simulink model "BuildingHeatLoadCalc"  (R2026a)
settings: Solver=ode1be  StopTime=31532400  FixedStep=3600  AbsTol=1e-3
undefined symbols (not defined in the file): BuildingThermalLib, lib_BuildingThermal
libraries: ExternalWall_lib x47, WallSelector_lib x36, fl_lib x32, RoomWithAirVolume x15, nesl_utility x4, TemperatureSource_lib x1, DayScheduler_lib x1, SolarRadiationAtLocation_lib x1
(part 1 of 5)
settings Model: Creator=vikrants  LastModifiedBy=vikrants
settings DebuggingCC: SymbolicDimsDataTypeCodeGenerationDiagnostic=none
settings SimscapeCC: SimscapeNominalValues="[{\"value\":\"1\",\"unit\":\"A\"},{\"value\":\"1\",\"unit\":\"bar\"},{\"value\":\"1\",\"unit\":\"cm^2\"},{\"value\":\"1\",\"unit\":\"cm^3/s\"},{\"value\":\"1\",\"unit\":\"kJ/kg\"},{\"value\":\"1\",\"unit\":\"kW\"},{\"value\":\"1\",\"unit\":\"l\"},{\"value\":\"1\",\"unit\":\"N\"},{\"value\":\"1\",\"unit\":\"N*m\"},{\"value\":\"1\",\"unit\":\"V\"}]"  SimscapeLogSimulationStatistics=on

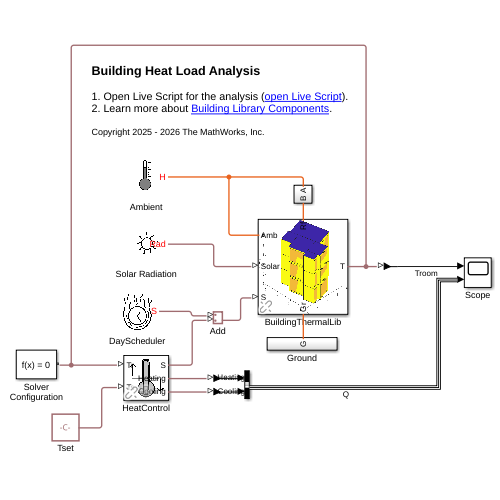
[thumbnail: Simulink's stored preview of the top-level diagram]
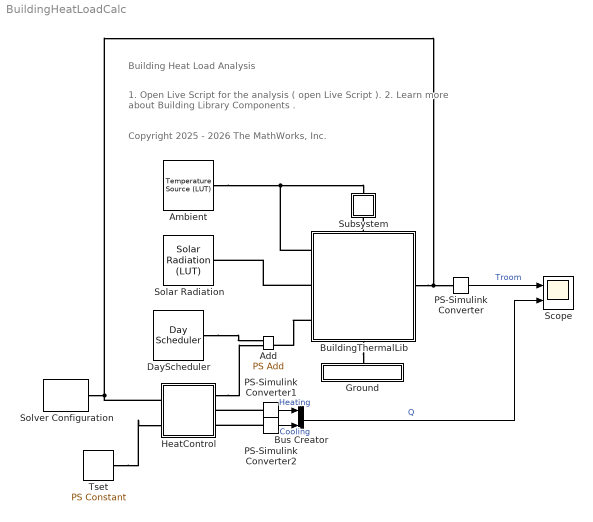
== system BuildingHeatLoadCalc ==
  note: Copyright 2025 - 2026 The MathWorks, Inc.
  note: Building Heat Load Analysis
  note: 1. Open Live Script for the analysis ( open Live Script ).
      | 2. Learn more about Building Library Components .
  Add : fl_lib/Physical Signals/Functions/PS Add
  Ambient : TemperatureSource_lib/Temperature Source (LUT)  latitude=47.376 % Parameterized on : 09-Jun-2026 19:38:28  longitude=8.541 % Parameterized on : 09-Jun-2026 19:38:29  localTime=15.00 % Parameterized on : 09-Jun-2026 19:38:29  dayLightS=0 % Parameterized on : 09-Jun-2026 19:38:29  startYear=2024 % Parameterized on : 09-Jun-2026 19:38:29  startMonth=1 % Parameterized on : 09-Jun-2026 19:38:29  startDay=1 % Parameterized on : 09-Jun-2026 19:38:29  startHr=1 % Parameterized on : 09-Jun-2026 19:38:29  numDaysData=365 % Parameterized on : 09-Jun-2026 19:38:29  interp_method=simscape.enum.interpolation.linear  extrap_method=simscape.enum.extrapolation.error  avgDayTvec="[275.3273      275.3222      275.3145      275.3043      275.2918      275.2771      275.3018      275.3282      275.3563      275.3861      275.4173        275.45      275.4841      275.5195      275.5562       275.594      275.6331      275.6733      275.7145      275.7568         275.8      275.8386      275.8744      275.9074      275.9378      275.9656       275.991      276.0141      276.0349      276.0536      276.0701      276.0846      276.0971      276.1078      276.1166      276.1236      276.1305      276.1619      276.1941      276.2271       276.261      276.2956      276.3309       276.367      276.4038      276.4412      276.4794      276.5181      276.5575      276.5975      276.6381      276.6792      276.7333       276.785      276.8342      276.9014      276.9656      277.0268      277.0851      277.1404      277.1927       277.242      277.2883      277.3317       277.372      277.4094      277.4438      277.4999       277.556      277.6119      277.6889      277.7686      277.8509      277.9359      278.0236       278.114       278.207      278.3028      278.4011      278.5022       278.606      278.7124      278.8297      278.9463      279.0624      279.1766      279.2694      279.3592      279.4459      279.5295      279.6101      279.6876      279.7621      279.8335      279.9018      279.9671      280.0294      280.0904      280.1795      280.2693      280.3596      280.4567      280.5571      280.6608      280.7677       280.878      280.9915      281.1083      281.2284      281.3518      281.4785      281.6085      281.7417      281.8694      281.9961      282.0985      282.1971      282.2917      282.3825      282.4693      282.5523      282.6313      282.7065      282.7778      282.8451      282.9086      282.9681      283.0238      283.1102       283.192      283.2729      283.3518      283.4287      283.5036      283.5765      283.6475      283.7164      283.7834      283.8484      283.9114      283.9724      284.0314      284.0885      284.1997      284.3147      284.4321      284.5312      284.6314      284.7328      284.8353       284.939      285.0438      285.1498      285.2569      285.3651      285.4745      285.5851      285.6968      285.8072      285.8771      285.9433      285.9937       286.043      286.0913      286.1386      286.1849      286.2303      286.2746       286.318      286.3603      286.4017       286.442      286.4814      286.5198      286.5795      286.6422      286.6832      286.7242      286.7654      286.8066      286.8479      286.8892      286.9307      286.9722      287.0138      287.0554      287.0972       287.139      287.1809      287.2213      287.2359      287.2392      287.2429      287.2469      287.2511      287.2557      287.2606      287.2658      287.2713      287.2771      287.2833      287.2897      287.2964      287.3034      287.3108      287.3141      287.3186      287.2947      287.2701      287.2447      287.2186      287.1917       287.164      287.1356      287.1063      287.0764      287.0456      287.0141      286.9819      286.9489      286.8969       286.842       286.793      286.7455      286.6993      286.6545      286.6111       286.569      286.5284      286.4891      286.4511      286.4146      286.3794      286.3456      286.3132      286.2703      286.2305      286.1593       286.092      286.0289      285.9698      285.9148      285.8638      285.8168      285.7739      285.7351      285.7003      285.6696      285.6429      285.6203      285.6009      285.5726      285.4907      285.4055      285.3171      285.2255      285.1307      285.0327      284.9315      284.8271      284.7194      284.6086      284.4945      284.3772      284.2567       284.133      283.9973      283.8627      283.7683      283.6776      283.5904      283.5067      283.4267      283.3502      283.2772      283.2078       283.142      283.0798      283.0212      282.9661      282.9145      282.8475      282.7818      282.6951      282.6058      282.5138 ...(+1106 chars)] % Parameterized on : 09-Jun-2026 19:38:29 K"  pcDayTvar=2 % Parameterized on : 09-Jun-2026 19:38:29  avgNightTvec="[270.3273      270.3222      270.3145      270.3043      270.2918      270.2771      270.3018      270.3282      270.3563      270.3861      270.4173        270.45      270.4841      270.5195      270.5562       270.594      270.6331      270.6733      270.7145      270.7568         270.8      270.8386      270.8744      270.9074      270.9378      270.9656       270.991      271.0141      271.0349      271.0536      271.0701      271.0846      271.0971      271.1078      271.1166      271.1236      271.1305      271.1619      271.1941      271.2271       271.261      271.2956      271.3309       271.367      271.4038      271.4412      271.4794      271.5181      271.5575      271.5975      271.6381      271.6792      271.7333       271.785      271.8342      271.9014      271.9656      272.0268      272.0851      272.1404      272.1927       272.242      272.2883      272.3317       272.372      272.4094      272.4438      272.4999       272.556      272.6119      272.6889      272.7686      272.8509      272.9359      273.0236       273.114       273.207      273.3028      273.4011      273.5022       273.606      273.7124      273.8297      273.9463      274.0624      274.1766      274.2694      274.3592      274.4459      274.5295      274.6101      274.6876      274.7621      274.8335      274.9018      274.9671      275.0294      275.0904      275.1795      275.2693      275.3596      275.4567      275.5571      275.6608      275.7677       275.878      275.9915      276.1083      276.2284      276.3518      276.4785      276.6085      276.7417      276.8694      276.9961      277.0985      277.1971      277.2917      277.3825      277.4693      277.5523      277.6313      277.7065      277.7778      277.8451      277.9086      277.9681      278.0238      278.1102       278.192      278.2729      278.3518      278.4287      278.5036      278.5765      278.6475      278.7164      278.7834      278.8484      278.9114      278.9724      279.0314      279.0885      279.1997      279.3147      279.4321      279.5312      279.6314      279.7328      279.8353       279.939      280.0438      280.1498      280.2569      280.3651      280.4745      280.5851      280.6968      280.8072      280.8771      280.9433      280.9937       281.043      281.0913      281.1386      281.1849      281.2303      281.2746       281.318      281.3603      281.4017       281.442      281.4814      281.5198      281.5795      281.6422      281.6832      281.7242      281.7654      281.8066      281.8479      281.8892      281.9307      281.9722      282.0138      282.0554      282.0972       282.139      282.1809      282.2213      282.2359      282.2392      282.2429      282.2469      282.2511      282.2557      282.2606      282.2658      282.2713      282.2771      282.2833      282.2897      282.2964      282.3034      282.3108      282.3141      282.3186      282.2947      282.2701      282.2447      282.2186      282.1917       282.164      282.1356      282.1063      282.0764      282.0456      282.0141      281.9819      281.9489      281.8969       281.842       281.793      281.7455      281.6993      281.6545      281.6111       281.569      281.5284      281.4891      281.4511      281.4146      281.3794      281.3456      281.3132      281.2703      281.2305      281.1593       281.092      281.0289      280.9698      280.9148      280.8638      280.8168      280.7739      280.7351      280.7003      280.6696      280.6429      280.6203      280.6009      280.5726      280.4907      280.4055      280.3171      280.2255      280.1307      280.0327      279.9315      279.8271      279.7194      279.6086      279.4945      279.3772      279.2567       279.133      278.9973      278.8627      278.7683      278.6776      278.5904      278.5067      278.4267      278.3502      278.2772      278.2078       278.142      278.0798      278.0212      277.9661      277.9145      277.8475      277.7818      277.6951      277.6058      277.5138 ...(+1106 chars)] % Parameterized on : 09-Jun-2026 19:38:29 K"  pcNightTvar=3 % Parameterized on : 09-Jun-2026 19:38:29
  BuildingThermalLib : Subsystem  AncestorBlock=lib_BuildingThermal/BuildingThermalLib
      settings: PortSchema="{\"entries\":[{\"content\":{\"sides\":[{\"content\":{\"connectorIds\":[\"LConn1\",\"LConn2\",\"LConn3\"]},\"type\":\"ConnectorPlacement.EquallySpacedRectSide\",\"uuid\":\"02f2e3a8-9f92-46e9-bc8d-cac18fd60cc5\"},{\"content\":{\"connectorIds\":[\"RConn1\"],\"side\":\"RIGHT\"},\"type\":\"ConnectorPlacement.EquallySpacedRectSide\",\"uuid\":\"8e7293df-d9e6-4251-9074-f41050b516bb\"},{\"content\":{\"connectorIds\":[\"LConn4\"],\"side\":\"TOP\"},\"type\":\"ConnectorPlacement.EquallySpacedRectSide\",\"uuid\":\"59004dc2-3d8b-47ae-86a8-cbcf5fc5c8f5\"},{\"content\":{\"connectorIds\":[\"RConn2\"],\"side\":\"BOTTOM\"},\"type\":\"ConnectorPlacement.EquallySpacedRectSide\",\"uuid\":\"040a7ff5-3de3-404c-857a-2e2aad7a1fa3\"}]},\"type\":\"ConnectorPlacement.EquallySpacedConnector\",\"uuid\":\"ad5b2bd3-ca1b-4c9b-b2dc-e1849bcec5d6\"}],\"packageUris\":[\"http://schema.mathworks.com/mf0/Connector/R2020b\"],\"version\":\"1.0\"}"
      mask Display: image('lib_BuildingThermal.png')
  Bus Creator : BusCreator  Inputs=2
  DayScheduler : DayScheduler_lib/Day Scheduler  numRoom=15 % Parameterized on : 09-Jun-2026 19:38:32  roomIndex=[1 2 3 4 5 6 7 8 9 10 11 12 13 14 15] % Parameterized on : 09-Jun-2026 19:38:32  heatSource=[0 0 0 0 0 0 0 0 0 0 0 0 0 0 0 0 0 0 0 0 0 0 0 0;200 200 200 200 200 200 0 0 0 0 0 0 0 0 0 0 0 0 0 200 200 200 200 200;0 0 0 0 0 300 300 0 0 0 0 0 0 0 0 0 0 300 300 300 300 0 0 0;0 0 0 0 0 0 0 0 0 0 0 0 0 0 0 0 0 0 0 0 0 0 0 0;0 0 0 0 0 0 0 0 0 0 0 0 0 0 0 0 0 0 0 0 0 0 0 0;0 0 0 0 0 0 0 0 0 0 0 0 0 0 0 0 0 0 0 0 0 0 0 0;200 200 200 200 200 200 0 0 0 0 0 0 0 0 0 0 0 0 0 200 200 200 200 200;0 0 0 0 0 300 300 0 0 0 0 0 0 0 0 0 0 300 300 300 300 0 0 0;0 0 0 0 0 0 0 0 0 0 0 0 0 0 0 0 0 0 0 0 0 0 0 0;0 0 0 0 0 0 0 0 0 0 0 0 0 0 0 0 0 0 0 0 0 0 0 0;0 0 0 0 0 0 0 0 0 0 0 0 0 0 0 0 0 0 0 0 0 0 0 0;200 200 200 200 200 200 0 0 0 0 0 0 0 0 0 0 0 0 0 200 200 200 200 200;0 0 0 0 0 300 300 0 0 0 0 0 0 0 0 0 0 300 300 300 300 0 0 0;0 0 0 0 0 0 0 0 0 0 0 0 0 0 0 0 0 0 0 0 0 0 0 0;0 0 0 0 0 0 0 0 0 0 0 0 0 0 0 0 0 0 0 0 0 0 0 0] % Parameterized on : 09-Jun-2026 19:38:32 W  t=1 : 24  oneHr=3600
  Ground : Subsystem
      settings: PortSchema="{\"entries\":[{\"content\":{\"sides\":[{\"content\":{},\"type\":\"ConnectorPlacement.EquallySpacedRectSide\",\"uuid\":\"0537d5ec-4a94-45e2-a0dd-9776fcfbef5c\"},{\"content\":{\"side\":\"RIGHT\"},\"type\":\"ConnectorPlacement.EquallySpacedRectSide\",\"uuid\":\"ea52c298-5a99-4146-b05a-e741d3f0a75b\"},{\"content\":{\"connectorIds\":[\"LConn1\"],\"side\":\"TOP\"},\"type\":\"ConnectorPlacement.EquallySpacedRectSide\",\"uuid\":\"d3185eb6-f3c0-4f94-b2cb-94c943d4e977\"}]},\"type\":\"ConnectorPlacement.EquallySpacedConnector\",\"uuid\":\"099be505-a3d7-43d0-9da6-14e4de4f60b9\"}],\"packageUris\":[\"http://schema.mathworks.com/mf0/Connector/R2020b\"],\"version\":\"1.0\"}"
  HeatControl : Subsystem  AncestorBlock=HeatSourceControl/Heat Source Control  mask{capacity=12000, num=3, delT=10, tau=1, iniT=280}
      mask prompts: capacity "Heat pump capacity (W)"; num "Number of sources (-)"; delT "Change in water temperature (deg C)"; tau "Measurement time constant (s)"; iniT "Initial water temperature (K)"
      mask DialogControl DescTextVar Prompt: Simple heat source pump based on temperature difference between measured and set point values. The pump is an abstract implementation for Air Water Heat Pump (AWHP).
      mask DialogControl HeatPump Prompt: Heat Pump
      mask Display: image('HeatSourceControlIcon.png');
  PS-Simulink Converter : nesl_utility/PS-Simulink Converter  PhysicalDomain=network_engine_domain  SubClassName=ps_output  LeftPortType=input  RightPortType=output  PseudoPeriodic=off  Frequencies=[]  VectorFormat=inherit  Unit=inherit  AffineConversion=off
  PS-Simulink Converter1 : nesl_utility/PS-Simulink Converter  PhysicalDomain=network_engine_domain  SubClassName=ps_output  LeftPortType=input  RightPortType=output  PseudoPeriodic=off  Frequencies=[]  VectorFormat=inherit  Unit=inherit  AffineConversion=off
  PS-Simulink Converter2 : nesl_utility/PS-Simulink Converter  PhysicalDomain=network_engine_domain  SubClassName=ps_output  LeftPortType=input  RightPortType=output  PseudoPeriodic=off  Frequencies=[]  VectorFormat=inherit  Unit=inherit  AffineConversion=off
  Scope : Scope  NumInputPorts=2
      settings: ActiveDisplayYMinimum=-1  ActiveDisplayYMaximum=1
  Solar Radiation : SolarRadiationAtLocation_lib/Solar Radiation (LUT)  latitude=47.376 % Parameterized on : 09-Jun-2026 19:38:30  longitude=8.541 % Parameterized on : 09-Jun-2026 19:38:30  localTime=15.00 % Parameterized on : 09-Jun-2026 19:38:30  dayLightS=0 % Parameterized on : 09-Jun-2026 19:38:31  startYear=2024 % Parameterized on : 09-Jun-2026 19:38:30  startMonth=1 % Parameterized on : 09-Jun-2026 19:38:31  startDay=1 % Parameterized on : 09-Jun-2026 19:38:31  startHr=1 % Parameterized on : 09-Jun-2026 19:38:31  numHrsData=8760 % Parameterized on : 09-Jun-2026 19:38:31  cloudData=cloudCoverLibOption.none  cloudCoverVal=zeros(1, 24)  interp_method=simscape.enum.interpolation.linear  extrap_method=simscape.enum.extrapolation.nearest
  Solver Configuration : nesl_utility/Solver Configuration  PhysicalDomain=network_engine_domain  SubClassName=solver  LeftPortType=input  RightPortType=generic  Tones=[]  Harmonics=[]  SimulateNoise=off  Profile=off  UseLocalSampling=off  EnableSwitchedLinearOptims=on  FrequencyDomain=off  UseCCode=off  RelTol=0.001  AbsTol=1e-06  MinStep=1e-09  ToWorkspace=off  RevertToSquareIcSolve=off  NumHomotopyIterations=100  PhasorMode=off  PhasorModeNumHarmonics=1  ConsistencySolver=NEWTON_XTOL_AFTER_FTOL  CanonicalOrdering=UNORDERED  OptimizeIntermediates=UNOPTIMIZED  IndexReductionMethod=DerivativeReplacement  DoDC=off  ResidualTolerance=1e-09  ConsistencyTolSource=GLOBAL  ConsistencyAbsTol=0.001  ConsistencyRelTol=0.001  ConsistencyTolFactor=0.001  UseLocalSolver=off  LocalSolverChoice=NE_BACKWARD_EULER_ADVANCER  ResolveIndetEquations=on  FunctionEvalNumThread=1  LocalSolverSampleTime=0.001  DoFixedCost=off  MaxNonlinIter=3  MaxModeIter=2  ComputeImpulses=off  ImpulseIterations=2  LinearAlgebra=auto  LinearAlgebraNumThread=0  EquationFormulation=NE_TIME_EF  DelaysMemoryBudget=1024  AutomaticFiltering=on  FilteringTimeConstant=0.001  PartitionStorageMethod=AS_NEEDED  PartitionMemoryBudget=1024  PartitionMethod=ROBUST  MultibodyUseLocalSolver=off  MultibodyLocalSolverChoice=ODE1  MultibodyLocalSolverSampleTime=0.001
  Subsystem : Subsystem
  Tset : fl_lib/Physical Signals/Sources/PS Constant  constant=293 % Parameterized on : 09-Jun-2026 19:38:32 K
  wires:
  PS-Simulink Converter/1 -> Scope/1  "Troom"
  PS-Simulink Converter2/1 -> Bus Creator/2  "Cooling"
  PS-Simulink Converter1/1 -> Bus Creator/1  "Heating"
  Bus Creator/1 -> Scope/2  "Q"
  connections:
  BuildingThermalLib/LConn2 -- Solar Radiation/RConn1
  BuildingThermalLib/LConn3 -- Add/RConn1
  DayScheduler/RConn1 -- Add/LConn1
  HeatControl/LConn3 -- Add/LConn2
  HeatControl/RConn2 -- Solver Configuration/RConn1 -- BuildingThermalLib/RConn1 -- PS-Simulink Converter/LConn1
  PS-Simulink Converter1/LConn1 -- HeatControl/LConn2
  PS-Simulink Converter2/LConn1 -- HeatControl/LConn1
  Tset/RConn1 -- HeatControl/RConn1
  BuildingThermalLib/RConn2 -- Ground/LConn1
  Ambient/RConn1 -- Subsystem/LConn1 -- BuildingThermalLib/LConn1
  BuildingThermalLib/LConn4 -- Subsystem/RConn1

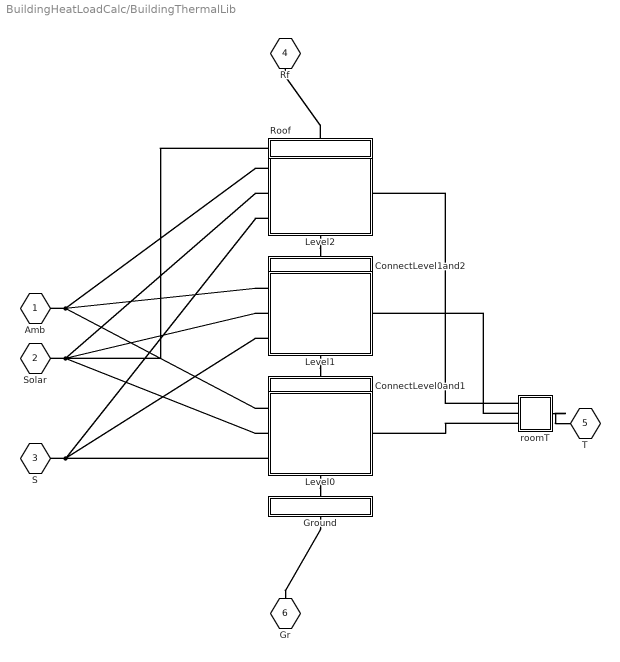
== system BuildingHeatLoadCalc/BuildingThermalLib ==
  ConnectLevel0and1 : Subsystem
      settings: PortSchema="{\"entries\":[{\"content\":{\"sides\":[{\"content\":{},\"type\":\"ConnectorPlacement.EquallySpacedRectSide\",\"uuid\":\"3fb70943-7938-4a07-9cd8-fdf0c154c089\"},{\"content\":{\"side\":\"RIGHT\"},\"type\":\"ConnectorPlacement.EquallySpacedRectSide\",\"uuid\":\"05a521c1-d6a1-4200-9b83-3d3259291215\"},{\"content\":{\"connectorIds\":[\"LConn1\"],\"side\":\"TOP\"},\"type\":\"ConnectorPlacement.EquallySpacedRectSide\",\"uuid\":\"456762b1-d32b-4bbd-9eba-67814e0f7e29\"},{\"content\":{\"connectorIds\":[\"RConn1\"],\"side\":\"BOTTOM\"},\"type\":\"ConnectorPlacement.EquallySpacedRectSide\",\"uuid\":\"1a1553e8-829a-4052-a1db-9258c9d2d2eb\"}]},\"type\":\"ConnectorPlacement.EquallySpacedConnector\",\"uuid\":\"0515c11f-813e-422f-b873-cfb943be20a0\"}],\"packageUris\":[\"http://schema.mathworks.com/mf0/Connector/R2020b\"],\"version\":\"1.0\"}"
  ConnectLevel1and2 : Subsystem
      settings: PortSchema="{\"entries\":[{\"content\":{\"sides\":[{\"content\":{},\"type\":\"ConnectorPlacement.EquallySpacedRectSide\",\"uuid\":\"3fb70943-7938-4a07-9cd8-fdf0c154c089\"},{\"content\":{\"side\":\"RIGHT\"},\"type\":\"ConnectorPlacement.EquallySpacedRectSide\",\"uuid\":\"05a521c1-d6a1-4200-9b83-3d3259291215\"},{\"content\":{\"connectorIds\":[\"LConn1\"],\"side\":\"TOP\"},\"type\":\"ConnectorPlacement.EquallySpacedRectSide\",\"uuid\":\"456762b1-d32b-4bbd-9eba-67814e0f7e29\"},{\"content\":{\"connectorIds\":[\"RConn1\"],\"side\":\"BOTTOM\"},\"type\":\"ConnectorPlacement.EquallySpacedRectSide\",\"uuid\":\"4a30b949-be85-43d7-93f8-e85595850486\"}]},\"type\":\"ConnectorPlacement.EquallySpacedConnector\",\"uuid\":\"0515c11f-813e-422f-b873-cfb943be20a0\"}],\"packageUris\":[\"http://schema.mathworks.com/mf0/Connector/R2020b\"],\"version\":\"1.0\"}"
  Ground : Subsystem
      settings: PortSchema="{\"entries\":[{\"content\":{\"sides\":[{\"content\":{},\"type\":\"ConnectorPlacement.EquallySpacedRectSide\",\"uuid\":\"3fb70943-7938-4a07-9cd8-fdf0c154c089\"},{\"content\":{\"side\":\"RIGHT\"},\"type\":\"ConnectorPlacement.EquallySpacedRectSide\",\"uuid\":\"05a521c1-d6a1-4200-9b83-3d3259291215\"},{\"content\":{\"connectorIds\":[\"LConn1\"],\"side\":\"TOP\"},\"type\":\"ConnectorPlacement.EquallySpacedRectSide\",\"uuid\":\"456762b1-d32b-4bbd-9eba-67814e0f7e29\"},{\"content\":{\"connectorIds\":[\"RConn1\"],\"side\":\"BOTTOM\"},\"type\":\"ConnectorPlacement.EquallySpacedRectSide\",\"uuid\":\"a4d2ba80-0adb-4d34-9370-eb9583c2211d\"}]},\"type\":\"ConnectorPlacement.EquallySpacedConnector\",\"uuid\":\"0515c11f-813e-422f-b873-cfb943be20a0\"}],\"packageUris\":[\"http://schema.mathworks.com/mf0/Connector/R2020b\"],\"version\":\"1.0\"}"
  Level0 : Subsystem
      settings: PortSchema="{\"entries\":[{\"content\":{\"sides\":[{\"content\":{\"connectorIds\":[\"LConn1\",\"LConn2\",\"LConn3\"]},\"type\":\"ConnectorPlacement.EquallySpacedRectSide\",\"uuid\":\"5074afe5-1eb3-4154-99f1-11d56108c9ad\"},{\"content\":{\"connectorIds\":[\"RConn1\"],\"side\":\"RIGHT\"},\"type\":\"ConnectorPlacement.EquallySpacedRectSide\",\"uuid\":\"e70542b5-eb54-43d5-a4ec-335ad714f0fc\"},{\"content\":{\"connectorIds\":[\"LConn4\"],\"side\":\"TOP\"},\"type\":\"ConnectorPlacement.EquallySpacedRectSide\",\"uuid\":\"d6546cf1-a767-41eb-8f4c-4906164cfa57\"},{\"content\":{\"connectorIds\":[\"RConn2\"],\"side\":\"BOTTOM\"},\"type\":\"ConnectorPlacement.EquallySpacedRectSide\",\"uuid\":\"8d7be69c-f27b-4abc-b500-3a84c55d47c4\"}]},\"type\":\"ConnectorPlacement.EquallySpacedConnector\",\"uuid\":\"ebb60fe0-0ae9-4e41-adc3-c2c3cb70ecfc\"}],\"packageUris\":[\"http://schema.mathworks.com/mf0/Connector/R2020b\"],\"version\":\"1.0\"}"
  Level1 : Subsystem
      settings: PortSchema="{\"entries\":[{\"content\":{\"sides\":[{\"content\":{\"connectorIds\":[\"LConn1\",\"LConn2\",\"LConn3\"]},\"type\":\"ConnectorPlacement.EquallySpacedRectSide\",\"uuid\":\"5074afe5-1eb3-4154-99f1-11d56108c9ad\"},{\"content\":{\"connectorIds\":[\"RConn1\"],\"side\":\"RIGHT\"},\"type\":\"ConnectorPlacement.EquallySpacedRectSide\",\"uuid\":\"e70542b5-eb54-43d5-a4ec-335ad714f0fc\"},{\"content\":{\"connectorIds\":[\"LConn4\"],\"side\":\"TOP\"},\"type\":\"ConnectorPlacement.EquallySpacedRectSide\",\"uuid\":\"d6546cf1-a767-41eb-8f4c-4906164cfa57\"},{\"content\":{\"connectorIds\":[\"RConn2\"],\"side\":\"BOTTOM\"},\"type\":\"ConnectorPlacement.EquallySpacedRectSide\",\"uuid\":\"0ce4d1e7-6fe2-4298-a820-c321d652306b\"}]},\"type\":\"ConnectorPlacement.EquallySpacedConnector\",\"uuid\":\"ebb60fe0-0ae9-4e41-adc3-c2c3cb70ecfc\"}],\"packageUris\":[\"http://schema.mathworks.com/mf0/Connector/R2020b\"],\"version\":\"1.0\"}"
  Level2 : Subsystem
      settings: PortSchema="{\"entries\":[{\"content\":{\"sides\":[{\"content\":{\"connectorIds\":[\"LConn1\",\"LConn2\",\"LConn3\"]},\"type\":\"ConnectorPlacement.EquallySpacedRectSide\",\"uuid\":\"5074afe5-1eb3-4154-99f1-11d56108c9ad\"},{\"content\":{\"connectorIds\":[\"RConn1\"],\"side\":\"RIGHT\"},\"type\":\"ConnectorPlacement.EquallySpacedRectSide\",\"uuid\":\"e70542b5-eb54-43d5-a4ec-335ad714f0fc\"},{\"content\":{\"connectorIds\":[\"LConn4\"],\"side\":\"TOP\"},\"type\":\"ConnectorPlacement.EquallySpacedRectSide\",\"uuid\":\"d6546cf1-a767-41eb-8f4c-4906164cfa57\"},{\"content\":{\"connectorIds\":[\"RConn2\"],\"side\":\"BOTTOM\"},\"type\":\"ConnectorPlacement.EquallySpacedRectSide\",\"uuid\":\"ae0b0ecc-8cea-42a6-9f86-a2fcc6949a4a\"}]},\"type\":\"ConnectorPlacement.EquallySpacedConnector\",\"uuid\":\"ebb60fe0-0ae9-4e41-adc3-c2c3cb70ecfc\"}],\"packageUris\":[\"http://schema.mathworks.com/mf0/Connector/R2020b\"],\"version\":\"1.0\"}"
  Roof : Subsystem
      settings: PortSchema="{\"entries\":[{\"content\":{\"sides\":[{\"content\":{\"connectorIds\":[\"LConn1\"]},\"type\":\"ConnectorPlacement.EquallySpacedRectSide\",\"uuid\":\"0be4c07b-4a16-48eb-ba1a-eb19140d6e21\"},{\"content\":{\"side\":\"RIGHT\"},\"type\":\"ConnectorPlacement.EquallySpacedRectSide\",\"uuid\":\"1d83c5b9-3651-480e-b537-4a87f3d8118d\"},{\"content\":{\"connectorIds\":[\"LConn2\"],\"side\":\"TOP\"},\"type\":\"ConnectorPlacement.EquallySpacedRectSide\",\"uuid\":\"3c581fde-8499-4f6e-8539-a668eefd365a\"},{\"content\":{\"connectorIds\":[\"RConn1\"],\"side\":\"BOTTOM\"},\"type\":\"ConnectorPlacement.EquallySpacedRectSide\",\"uuid\":\"56c2556b-374c-4a46-bad4-c741fb2c6272\"}]},\"type\":\"ConnectorPlacement.EquallySpacedConnector\",\"uuid\":\"dfabb703-80b0-43fd-81cb-1196e1f2c066\"}],\"packageUris\":[\"http://schema.mathworks.com/mf0/Connector/R2020b\"],\"version\":\"1.0\"}"
  roomT : Subsystem
  Amb : PMIOPort  Side=Left
  Solar : PMIOPort  Port=2  Side=Left
  S : PMIOPort  Port=3  Side=Left
  Rf : PMIOPort  Port=4  Side=Left
  T : PMIOPort  Port=5  Side=Right
  Gr : PMIOPort  Port=6  Side=Right
  connections:
  Level0/RConn2 -- Ground/LConn1
  Level1/RConn2 -- ConnectLevel0and1/LConn1
  Level0/LConn4 -- ConnectLevel0and1/RConn1
  Level2/RConn2 -- ConnectLevel1and2/LConn1
  Level1/LConn4 -- ConnectLevel1and2/RConn1
  Level2/LConn4 -- Roof/RConn1
  Roof/LConn2 -- Rf/RConn1
  Ground/RConn1 -- Gr/RConn1
  Roof/LConn1 -- Level0/LConn2 -- Level1/LConn2 -- Solar/RConn1 -- Level2/LConn2
  Level0/LConn1 -- Level1/LConn1 -- Amb/RConn1 -- Level2/LConn1
  Level0/LConn3 -- Level1/LConn3 -- S/RConn1 -- Level2/LConn3
  roomT/LConn1 -- Level2/RConn1
  roomT/LConn2 -- Level1/RConn1
  roomT/LConn3 -- Level0/RConn1
  roomT/RConn1 -- T/RConn1

== system BuildingHeatLoadCalc/Ground ==
  Array Connection1 : SimscapeArrayConnection  Domain=foundation.thermal.thermal  ConcatenateDimension=1  NumScalarElements=5
  Perfect Insulator{,1..4} (5 alike) : fl_lib/Thermal/Thermal Elements/Perfect Insulator  T_specify=off  T_priority=None  T=293.15 K  T_nominal_specify=off  T_nominal_value=1  T_nominal_unit=K
  G : PMIOPort  Side=Left
  connections:
  Perfect Insulator3/LConn1 -- Array Connection1/LConn3
  Perfect Insulator4/LConn1 -- Array Connection1/LConn2
  Perfect Insulator2/LConn1 -- Array Connection1/LConn4
  Perfect Insulator1/LConn1 -- Array Connection1/LConn5
  Perfect Insulator/LConn1 -- Array Connection1/LConn1
  Array Connection1/RConn1 -- G/RConn1

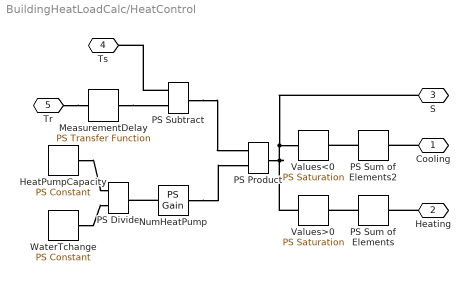
== system BuildingHeatLoadCalc/HeatControl ==
  HeatPumpCapacity : fl_lib/Physical Signals/Sources/PS Constant  constant=capacity J/s
  MeasurementDelay : fl_lib/Physical Signals/Linear Operators/PS Transfer Function  transfer_function_type=foundation.enum.transfer_function_type.lag  T=tau s  T1=2 s  T2=1 s  reset_method=foundation.enum.IntegratorResetSpec.None  initial_condition_spec=foundation.enum.IntegratorICSpec.Internal  y0=iniT K
  NumHeatPump : fl_lib/Physical Signals/Functions/PS Gain  gain=num
  PS Divide : fl_lib/Physical Signals/Functions/PS Divide
  PS Product : fl_lib/Physical Signals/Functions/PS Product
  PS Subtract : fl_lib/Physical Signals/Functions/PS Subtract
  PS Sum of Elements : fl_lib/Physical Signals/Functions/PS Sum of Elements  sumAll=true
  PS Sum of Elements2 : fl_lib/Physical Signals/Functions/PS Sum of Elements  sumAll=true
  Values<0 : fl_lib/Physical Signals/Nonlinear Operators/PS Saturation  upper_limit=0 J/s  lower_limit=-inf J/s  ZeroCross=true
  Values>0 : fl_lib/Physical Signals/Nonlinear Operators/PS Saturation  upper_limit=inf J/s  lower_limit=0 J/s  ZeroCross=true
  WaterTchange : fl_lib/Physical Signals/Sources/PS Constant  constant=delT K
  Cooling : PMIOPort  Side=Left
  Heating : PMIOPort  Port=2  Side=Left
  S : PMIOPort  Port=3  Side=Left
  Ts : PMIOPort  Port=4  Side=Right
  Tr : PMIOPort  Port=5  Side=Right
  connections:
  PS Product/RConn1 -- Values>0/LConn1 -- Values<0/LConn1 -- S/RConn1
  NumHeatPump/RConn1 -- PS Product/LConn2
  NumHeatPump/LConn1 -- PS Divide/RConn1
  WaterTchange/RConn1 -- PS Divide/LConn2
  HeatPumpCapacity/RConn1 -- PS Divide/LConn1
  MeasurementDelay/RConn1 -- PS Subtract/LConn2
  PS Sum of Elements2/LConn1 -- Values<0/RConn1
  PS Sum of Elements/LConn1 -- Values>0/RConn1
  Cooling/RConn1 -- PS Sum of Elements2/RConn1
  Heating/RConn1 -- PS Sum of Elements/RConn1
  PS Subtract/LConn1 -- Ts/RConn1
  Tr/RConn1 -- MeasurementDelay/LConn1
  PS Subtract/RConn1 -- PS Product/LConn1

== system BuildingHeatLoadCalc/Subsystem ==
  Array Connection : SimscapeArrayConnection  Domain=foundation.thermal.thermal  ConcatenateDimension=1  NumScalarElements=5
  A : PMIOPort  Side=Left
  B : PMIOPort  Port=2  Side=Right
  connections:
  Array Connection/LConn1 -- A/RConn1 -- Array Connection/LConn4 -- Array Connection/LConn5 -- Array Connection/LConn3 -- Array Connection/LConn2
  B/RConn1 -- Array Connection/RConn1

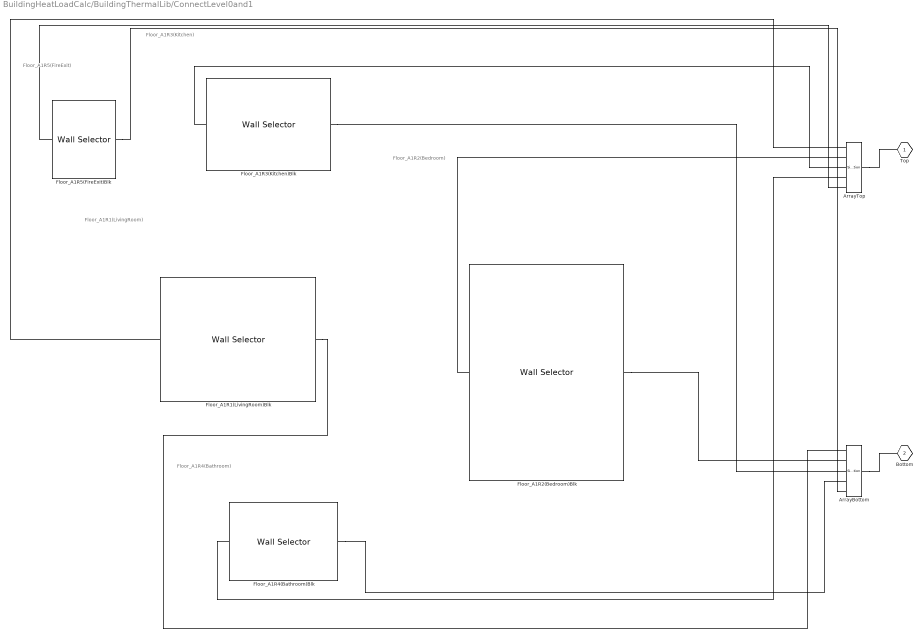
== system BuildingHeatLoadCalc/BuildingThermalLib/ConnectLevel0and1 ==
  note: Floor_A1R1(LivingRoom)
  note: Floor_A1R2(Bedroom)
  note: Floor_A1R3(Kitchen)
  note: Floor_A1R4(Bathroom)
  note: Floor_A1R5(FireExit)
  ArrayBottom : SimscapeArrayConnection  Domain=foundation.thermal.thermal  ConcatenateDimension=1  NumScalarElements=5
  ArrayTop : SimscapeArrayConnection  Domain=foundation.thermal.thermal  ConcatenateDimension=1  NumScalarElements=5
  Floor_A1R1(LivingRoom)Blk : WallSelector_lib/Wall Selector  optWall=wallModelOption.wallOnly  wallLength=2.4384 % Parameterized on : 09-Jun-2026 19:35:13 m  wallHeight=3.048 % Parameterized on : 09-Jun-2026 19:35:13 m  wallThickness=0.03 % Parameterized on : 09-Jun-2026 19:35:13 m  wallMaterialDen=1400 % Parameterized on : 09-Jun-2026 19:35:15 kg/m^3  wallMaterialCp=1000 % Parameterized on : 09-Jun-2026 19:35:15 J/(K*kg)  wallAbsorptivity=0.5  wallThermalK=0.7 % Parameterized on : 09-Jun-2026 19:35:15 W/(K*m)  winLength=1 m  winHeight=0.5 m  winThickness=0.007 m  winMaterialDen=2500 kg/m^3  winMaterialCp=787 J/(K*kg)  winAbsorptivity=0.35  winThermalK=1 W/(K*m)  winTransmissivity=0.45  ventLength=0.1 m  ventHeight=0.1 m  extToWallHTC=30 % Parameterized on : 09-Jun-2026 19:35:15 W/(K*m^2)  intToRoomHTC=30 % Parameterized on : 09-Jun-2026 19:35:15 W/(K*m^2)  iniT=275.8 % Parameterized on : 09-Jun-2026 19:38:28 K
  Floor_A1R2(Bedroom)Blk : WallSelector_lib/Wall Selector  optWall=wallModelOption.wallOnly  wallLength=4.2672 % Parameterized on : 09-Jun-2026 19:35:13 m  wallHeight=3.048 % Parameterized on : 09-Jun-2026 19:35:13 m  wallThickness=0.03 % Parameterized on : 09-Jun-2026 19:35:13 m  wallMaterialDen=1400 % Parameterized on : 09-Jun-2026 19:35:15 kg/m^3  wallMaterialCp=1000 % Parameterized on : 09-Jun-2026 19:35:15 J/(K*kg)  wallAbsorptivity=0.5  wallThermalK=0.7 % Parameterized on : 09-Jun-2026 19:35:15 W/(K*m)  winLength=1 m  winHeight=0.5 m  winThickness=0.007 m  winMaterialDen=2500 kg/m^3  winMaterialCp=787 J/(K*kg)  winAbsorptivity=0.35  winThermalK=1 W/(K*m)  winTransmissivity=0.45  ventLength=0.1 m  ventHeight=0.1 m  extToWallHTC=30 % Parameterized on : 09-Jun-2026 19:35:15 W/(K*m^2)  intToRoomHTC=30 % Parameterized on : 09-Jun-2026 19:35:15 W/(K*m^2)  iniT=275.8 % Parameterized on : 09-Jun-2026 19:38:28 K
  Floor_A1R3(Kitchen)Blk : WallSelector_lib/Wall Selector  optWall=wallModelOption.wallOnly  wallLength=1.8288 % Parameterized on : 09-Jun-2026 19:35:13 m  wallHeight=2.4384 % Parameterized on : 09-Jun-2026 19:35:13 m  wallThickness=0.03 % Parameterized on : 09-Jun-2026 19:35:13 m  wallMaterialDen=1400 % Parameterized on : 09-Jun-2026 19:35:15 kg/m^3  wallMaterialCp=1000 % Parameterized on : 09-Jun-2026 19:35:15 J/(K*kg)  wallAbsorptivity=0.5  wallThermalK=0.7 % Parameterized on : 09-Jun-2026 19:35:15 W/(K*m)  winLength=1 m  winHeight=0.5 m  winThickness=0.007 m  winMaterialDen=2500 kg/m^3  winMaterialCp=787 J/(K*kg)  winAbsorptivity=0.35  winThermalK=1 W/(K*m)  winTransmissivity=0.45  ventLength=0.1 m  ventHeight=0.1 m  extToWallHTC=30 % Parameterized on : 09-Jun-2026 19:35:15 W/(K*m^2)  intToRoomHTC=30 % Parameterized on : 09-Jun-2026 19:35:15 W/(K*m^2)  iniT=275.8 % Parameterized on : 09-Jun-2026 19:38:28 K
  Floor_A1R4(Bathroom)Blk : WallSelector_lib/Wall Selector  optWall=wallModelOption.wallOnly  wallLength=1.524 % Parameterized on : 09-Jun-2026 19:35:13 m  wallHeight=2.1336 % Parameterized on : 09-Jun-2026 19:35:13 m  wallThickness=0.03 % Parameterized on : 09-Jun-2026 19:35:13 m  wallMaterialDen=1400 % Parameterized on : 09-Jun-2026 19:35:15 kg/m^3  wallMaterialCp=1000 % Parameterized on : 09-Jun-2026 19:35:15 J/(K*kg)  wallAbsorptivity=0.5  wallThermalK=0.7 % Parameterized on : 09-Jun-2026 19:35:15 W/(K*m)  winLength=1 m  winHeight=0.5 m  winThickness=0.007 m  winMaterialDen=2500 kg/m^3  winMaterialCp=787 J/(K*kg)  winAbsorptivity=0.35  winThermalK=1 W/(K*m)  winTransmissivity=0.45  ventLength=0.1 m  ventHeight=0.1 m  extToWallHTC=30 % Parameterized on : 09-Jun-2026 19:35:15 W/(K*m^2)  intToRoomHTC=30 % Parameterized on : 09-Jun-2026 19:35:15 W/(K*m^2)  iniT=275.8 % Parameterized on : 09-Jun-2026 19:38:28 K
  Floor_A1R5(FireExit)Blk : WallSelector_lib/Wall Selector  optWall=wallModelOption.wallOnly  wallLength=1.524 % Parameterized on : 09-Jun-2026 19:35:13 m  wallHeight=1.2192 % Parameterized on : 09-Jun-2026 19:35:13 m  wallThickness=0.03 % Parameterized on : 09-Jun-2026 19:35:13 m  wallMaterialDen=1400 % Parameterized on : 09-Jun-2026 19:35:15 kg/m^3  wallMaterialCp=1000 % Parameterized on : 09-Jun-2026 19:35:15 J/(K*kg)  wallAbsorptivity=0.5  wallThermalK=0.7 % Parameterized on : 09-Jun-2026 19:35:15 W/(K*m)  winLength=1 m  winHeight=0.5 m  winThickness=0.007 m  winMaterialDen=2500 kg/m^3  winMaterialCp=787 J/(K*kg)  winAbsorptivity=0.35  winThermalK=1 W/(K*m)  winTransmissivity=0.45  ventLength=0.1 m  ventHeight=0.1 m  extToWallHTC=30 % Parameterized on : 09-Jun-2026 19:35:15 W/(K*m^2)  intToRoomHTC=30 % Parameterized on : 09-Jun-2026 19:35:15 W/(K*m^2)  iniT=275.8 % Parameterized on : 09-Jun-2026 19:38:28 K
  Top : PMIOPort  Side=Left
  Bottom : PMIOPort  Port=2  Side=Right
  connections:
  ArrayTop/RConn1 -- Top/RConn1
  Floor_A1R1(LivingRoom)Blk/LConn1 -- ArrayTop/LConn1
  Floor_A1R2(Bedroom)Blk/LConn1 -- ArrayTop/LConn2
  Floor_A1R3(Kitchen)Blk/LConn1 -- ArrayTop/LConn3
  Floor_A1R4(Bathroom)Blk/LConn1 -- ArrayTop/LConn4
  Floor_A1R5(FireExit)Blk/LConn1 -- ArrayTop/LConn5
  ArrayBottom/RConn1 -- Bottom/RConn1
  Floor_A1R1(LivingRoom)Blk/RConn1 -- ArrayBottom/LConn1
  Floor_A1R2(Bedroom)Blk/RConn1 -- ArrayBottom/LConn2
  Floor_A1R3(Kitchen)Blk/RConn1 -- ArrayBottom/LConn3
  Floor_A1R4(Bathroom)Blk/RConn1 -- ArrayBottom/LConn4
  Floor_A1R5(FireExit)Blk/RConn1 -- ArrayBottom/LConn5

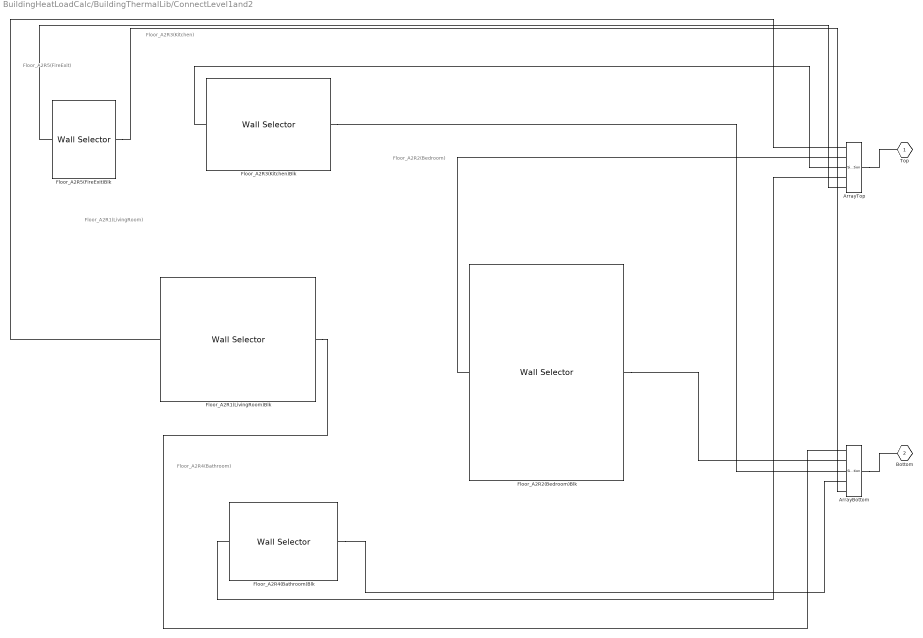
== system BuildingHeatLoadCalc/BuildingThermalLib/ConnectLevel1and2 ==
  note: Floor_A2R1(LivingRoom)
  note: Floor_A2R2(Bedroom)
  note: Floor_A2R3(Kitchen)
  note: Floor_A2R4(Bathroom)
  note: Floor_A2R5(FireExit)
  ArrayBottom : SimscapeArrayConnection  Domain=foundation.thermal.thermal  ConcatenateDimension=1  NumScalarElements=5
  ArrayTop : SimscapeArrayConnection  Domain=foundation.thermal.thermal  ConcatenateDimension=1  NumScalarElements=5
  Floor_A2R1(LivingRoom)Blk : WallSelector_lib/Wall Selector  optWall=wallModelOption.wallOnly  wallLength=2.4384 % Parameterized on : 09-Jun-2026 19:35:13 m  wallHeight=3.048 % Parameterized on : 09-Jun-2026 19:35:13 m  wallThickness=0.03 % Parameterized on : 09-Jun-2026 19:35:13 m  wallMaterialDen=1400 % Parameterized on : 09-Jun-2026 19:35:15 kg/m^3  wallMaterialCp=1000 % Parameterized on : 09-Jun-2026 19:35:15 J/(K*kg)  wallAbsorptivity=0.5  wallThermalK=0.7 % Parameterized on : 09-Jun-2026 19:35:15 W/(K*m)  winLength=1 m  winHeight=0.5 m  winThickness=0.007 m  winMaterialDen=2500 kg/m^3  winMaterialCp=787 J/(K*kg)  winAbsorptivity=0.35  winThermalK=1 W/(K*m)  winTransmissivity=0.45  ventLength=0.1 m  ventHeight=0.1 m  extToWallHTC=30 % Parameterized on : 09-Jun-2026 19:35:15 W/(K*m^2)  intToRoomHTC=30 % Parameterized on : 09-Jun-2026 19:35:15 W/(K*m^2)  iniT=275.8 % Parameterized on : 09-Jun-2026 19:38:28 K
  Floor_A2R2(Bedroom)Blk : WallSelector_lib/Wall Selector  optWall=wallModelOption.wallOnly  wallLength=4.2672 % Parameterized on : 09-Jun-2026 19:35:13 m  wallHeight=3.048 % Parameterized on : 09-Jun-2026 19:35:13 m  wallThickness=0.03 % Parameterized on : 09-Jun-2026 19:35:13 m  wallMaterialDen=1400 % Parameterized on : 09-Jun-2026 19:35:15 kg/m^3  wallMaterialCp=1000 % Parameterized on : 09-Jun-2026 19:35:15 J/(K*kg)  wallAbsorptivity=0.5  wallThermalK=0.7 % Parameterized on : 09-Jun-2026 19:35:15 W/(K*m)  winLength=1 m  winHeight=0.5 m  winThickness=0.007 m  winMaterialDen=2500 kg/m^3  winMaterialCp=787 J/(K*kg)  winAbsorptivity=0.35  winThermalK=1 W/(K*m)  winTransmissivity=0.45  ventLength=0.1 m  ventHeight=0.1 m  extToWallHTC=30 % Parameterized on : 09-Jun-2026 19:35:15 W/(K*m^2)  intToRoomHTC=30 % Parameterized on : 09-Jun-2026 19:35:15 W/(K*m^2)  iniT=275.8 % Parameterized on : 09-Jun-2026 19:38:28 K
  Floor_A2R3(Kitchen)Blk : WallSelector_lib/Wall Selector  optWall=wallModelOption.wallOnly  wallLength=1.8288 % Parameterized on : 09-Jun-2026 19:35:13 m  wallHeight=2.4384 % Parameterized on : 09-Jun-2026 19:35:13 m  wallThickness=0.03 % Parameterized on : 09-Jun-2026 19:35:13 m  wallMaterialDen=1400 % Parameterized on : 09-Jun-2026 19:35:15 kg/m^3  wallMaterialCp=1000 % Parameterized on : 09-Jun-2026 19:35:15 J/(K*kg)  wallAbsorptivity=0.5  wallThermalK=0.7 % Parameterized on : 09-Jun-2026 19:35:15 W/(K*m)  winLength=1 m  winHeight=0.5 m  winThickness=0.007 m  winMaterialDen=2500 kg/m^3  winMaterialCp=787 J/(K*kg)  winAbsorptivity=0.35  winThermalK=1 W/(K*m)  winTransmissivity=0.45  ventLength=0.1 m  ventHeight=0.1 m  extToWallHTC=30 % Parameterized on : 09-Jun-2026 19:35:15 W/(K*m^2)  intToRoomHTC=30 % Parameterized on : 09-Jun-2026 19:35:15 W/(K*m^2)  iniT=275.8 % Parameterized on : 09-Jun-2026 19:38:28 K
  Floor_A2R4(Bathroom)Blk : WallSelector_lib/Wall Selector  optWall=wallModelOption.wallOnly  wallLength=1.524 % Parameterized on : 09-Jun-2026 19:35:13 m  wallHeight=2.1336 % Parameterized on : 09-Jun-2026 19:35:13 m  wallThickness=0.03 % Parameterized on : 09-Jun-2026 19:35:13 m  wallMaterialDen=1400 % Parameterized on : 09-Jun-2026 19:35:15 kg/m^3  wallMaterialCp=1000 % Parameterized on : 09-Jun-2026 19:35:15 J/(K*kg)  wallAbsorptivity=0.5  wallThermalK=0.7 % Parameterized on : 09-Jun-2026 19:35:15 W/(K*m)  winLength=1 m  winHeight=0.5 m  winThickness=0.007 m  winMaterialDen=2500 kg/m^3  winMaterialCp=787 J/(K*kg)  winAbsorptivity=0.35  winThermalK=1 W/(K*m)  winTransmissivity=0.45  ventLength=0.1 m  ventHeight=0.1 m  extToWallHTC=30 % Parameterized on : 09-Jun-2026 19:35:15 W/(K*m^2)  intToRoomHTC=30 % Parameterized on : 09-Jun-2026 19:35:15 W/(K*m^2)  iniT=275.8 % Parameterized on : 09-Jun-2026 19:38:28 K
  Floor_A2R5(FireExit)Blk : WallSelector_lib/Wall Selector  optWall=wallModelOption.wallOnly  wallLength=1.524 % Parameterized on : 09-Jun-2026 19:35:13 m  wallHeight=1.2192 % Parameterized on : 09-Jun-2026 19:35:13 m  wallThickness=0.03 % Parameterized on : 09-Jun-2026 19:35:13 m  wallMaterialDen=1400 % Parameterized on : 09-Jun-2026 19:35:15 kg/m^3  wallMaterialCp=1000 % Parameterized on : 09-Jun-2026 19:35:15 J/(K*kg)  wallAbsorptivity=0.5  wallThermalK=0.7 % Parameterized on : 09-Jun-2026 19:35:15 W/(K*m)  winLength=1 m  winHeight=0.5 m  winThickness=0.007 m  winMaterialDen=2500 kg/m^3  winMaterialCp=787 J/(K*kg)  winAbsorptivity=0.35  winThermalK=1 W/(K*m)  winTransmissivity=0.45  ventLength=0.1 m  ventHeight=0.1 m  extToWallHTC=30 % Parameterized on : 09-Jun-2026 19:35:15 W/(K*m^2)  intToRoomHTC=30 % Parameterized on : 09-Jun-2026 19:35:15 W/(K*m^2)  iniT=275.8 % Parameterized on : 09-Jun-2026 19:38:28 K
  Top : PMIOPort  Side=Left
  Bottom : PMIOPort  Port=2  Side=Right
  connections:
  ArrayTop/RConn1 -- Top/RConn1
  Floor_A2R1(LivingRoom)Blk/LConn1 -- ArrayTop/LConn1
  Floor_A2R2(Bedroom)Blk/LConn1 -- ArrayTop/LConn2
  Floor_A2R3(Kitchen)Blk/LConn1 -- ArrayTop/LConn3
  Floor_A2R4(Bathroom)Blk/LConn1 -- ArrayTop/LConn4
  Floor_A2R5(FireExit)Blk/LConn1 -- ArrayTop/LConn5
  ArrayBottom/RConn1 -- Bottom/RConn1
  Floor_A2R1(LivingRoom)Blk/RConn1 -- ArrayBottom/LConn1
  Floor_A2R2(Bedroom)Blk/RConn1 -- ArrayBottom/LConn2
  Floor_A2R3(Kitchen)Blk/RConn1 -- ArrayBottom/LConn3
  Floor_A2R4(Bathroom)Blk/RConn1 -- ArrayBottom/LConn4
  Floor_A2R5(FireExit)Blk/RConn1 -- ArrayBottom/LConn5

== system BuildingHeatLoadCalc/BuildingThermalLib/Ground ==
  note: Ground_A1R1(LivingRoom)
  note: Ground_A1R2(Bedroom)
  note: Ground_A1R3(Kitchen)
  note: Ground_A1R4(Bathroom)
  note: Ground_A1R5(FireExit)
  ArrayBottom : SimscapeArrayConnection  Domain=foundation.thermal.thermal  ConcatenateDimension=1  NumScalarElements=5
  ArrayTop : SimscapeArrayConnection  Domain=foundation.thermal.thermal  ConcatenateDimension=1  NumScalarElements=5
  Ground_A1R1(LivingRoom)Blk : WallSelector_lib/Wall Selector  optWall=wallModelOption.wallOnly  wallLength=2.4384 % Parameterized on : 09-Jun-2026 19:35:13 m  wallHeight=3.048 % Parameterized on : 09-Jun-2026 19:35:13 m  wallThickness=0.03 % Parameterized on : 09-Jun-2026 19:35:13 m  wallMaterialDen=1400 % Parameterized on : 09-Jun-2026 19:35:15 kg/m^3  wallMaterialCp=1000 % Parameterized on : 09-Jun-2026 19:35:15 J/(K*kg)  wallAbsorptivity=0.5  wallThermalK=0.7 % Parameterized on : 09-Jun-2026 19:35:15 W/(K*m)  winLength=1 m  winHeight=0.5 m  winThickness=0.007 m  winMaterialDen=2500 kg/m^3  winMaterialCp=787 J/(K*kg)  winAbsorptivity=0.35  winThermalK=1 W/(K*m)  winTransmissivity=0.45  ventLength=0.1 m  ventHeight=0.1 m  extToWallHTC=30 % Parameterized on : 09-Jun-2026 19:35:15 W/(K*m^2)  intToRoomHTC=30 % Parameterized on : 09-Jun-2026 19:35:15 W/(K*m^2)  iniT=275.8 % Parameterized on : 09-Jun-2026 19:38:28 K
  Ground_A1R2(Bedroom)Blk : WallSelector_lib/Wall Selector  optWall=wallModelOption.wallOnly  wallLength=4.2672 % Parameterized on : 09-Jun-2026 19:35:13 m  wallHeight=3.048 % Parameterized on : 09-Jun-2026 19:35:13 m  wallThickness=0.03 % Parameterized on : 09-Jun-2026 19:35:13 m  wallMaterialDen=1400 % Parameterized on : 09-Jun-2026 19:35:15 kg/m^3  wallMaterialCp=1000 % Parameterized on : 09-Jun-2026 19:35:15 J/(K*kg)  wallAbsorptivity=0.5  wallThermalK=0.7 % Parameterized on : 09-Jun-2026 19:35:16 W/(K*m)  winLength=1 m  winHeight=0.5 m  winThickness=0.007 m  winMaterialDen=2500 kg/m^3  winMaterialCp=787 J/(K*kg)  winAbsorptivity=0.35  winThermalK=1 W/(K*m)  winTransmissivity=0.45  ventLength=0.1 m  ventHeight=0.1 m  extToWallHTC=30 % Parameterized on : 09-Jun-2026 19:35:16 W/(K*m^2)  intToRoomHTC=30 % Parameterized on : 09-Jun-2026 19:35:16 W/(K*m^2)  iniT=275.8 % Parameterized on : 09-Jun-2026 19:38:28 K
  Ground_A1R3(Kitchen)Blk : WallSelector_lib/Wall Selector  optWall=wallModelOption.wallOnly  wallLength=1.8288 % Parameterized on : 09-Jun-2026 19:35:13 m  wallHeight=2.4384 % Parameterized on : 09-Jun-2026 19:35:13 m  wallThickness=0.03 % Parameterized on : 09-Jun-2026 19:35:13 m  wallMaterialDen=1400 % Parameterized on : 09-Jun-2026 19:35:16 kg/m^3  wallMaterialCp=1000 % Parameterized on : 09-Jun-2026 19:35:16 J/(K*kg)  wallAbsorptivity=0.5  wallThermalK=0.7 % Parameterized on : 09-Jun-2026 19:35:16 W/(K*m)  winLength=1 m  winHeight=0.5 m  winThickness=0.007 m  winMaterialDen=2500 kg/m^3  winMaterialCp=787 J/(K*kg)  winAbsorptivity=0.35  winThermalK=1 W/(K*m)  winTransmissivity=0.45  ventLength=0.1 m  ventHeight=0.1 m  extToWallHTC=30 % Parameterized on : 09-Jun-2026 19:35:16 W/(K*m^2)  intToRoomHTC=30 % Parameterized on : 09-Jun-2026 19:35:16 W/(K*m^2)  iniT=275.8 % Parameterized on : 09-Jun-2026 19:38:28 K
  Ground_A1R4(Bathroom)Blk : WallSelector_lib/Wall Selector  optWall=wallModelOption.wallOnly  wallLength=1.524 % Parameterized on : 09-Jun-2026 19:35:13 m  wallHeight=2.1336 % Parameterized on : 09-Jun-2026 19:35:13 m  wallThickness=0.03 % Parameterized on : 09-Jun-2026 19:35:13 m  wallMaterialDen=1400 % Parameterized on : 09-Jun-2026 19:35:16 kg/m^3  wallMaterialCp=1000 % Parameterized on : 09-Jun-2026 19:35:16 J/(K*kg)  wallAbsorptivity=0.5  wallThermalK=0.7 % Parameterized on : 09-Jun-2026 19:35:16 W/(K*m)  winLength=1 m  winHeight=0.5 m  winThickness=0.007 m  winMaterialDen=2500 kg/m^3  winMaterialCp=787 J/(K*kg)  winAbsorptivity=0.35  winThermalK=1 W/(K*m)  winTransmissivity=0.45  ventLength=0.1 m  ventHeight=0.1 m  extToWallHTC=30 % Parameterized on : 09-Jun-2026 19:35:16 W/(K*m^2)  intToRoomHTC=30 % Parameterized on : 09-Jun-2026 19:35:16 W/(K*m^2)  iniT=275.8 % Parameterized on : 09-Jun-2026 19:38:28 K
  Ground_A1R5(FireExit)Blk : WallSelector_lib/Wall Selector  optWall=wallModelOption.wallOnly  wallLength=1.524 % Parameterized on : 09-Jun-2026 19:35:13 m  wallHeight=1.2192 % Parameterized on : 09-Jun-2026 19:35:13 m  wallThickness=0.03 % Parameterized on : 09-Jun-2026 19:35:13 m  wallMaterialDen=1400 % Parameterized on : 09-Jun-2026 19:35:16 kg/m^3  wallMaterialCp=1000 % Parameterized on : 09-Jun-2026 19:35:16 J/(K*kg)  wallAbsorptivity=0.5  wallThermalK=0.7 % Parameterized on : 09-Jun-2026 19:35:16 W/(K*m)  winLength=1 m  winHeight=0.5 m  winThickness=0.007 m  winMaterialDen=2500 kg/m^3  winMaterialCp=787 J/(K*kg)  winAbsorptivity=0.35  winThermalK=1 W/(K*m)  winTransmissivity=0.45  ventLength=0.1 m  ventHeight=0.1 m  extToWallHTC=30 % Parameterized on : 09-Jun-2026 19:35:16 W/(K*m^2)  intToRoomHTC=30 % Parameterized on : 09-Jun-2026 19:35:16 W/(K*m^2)  iniT=275.8 % Parameterized on : 09-Jun-2026 19:38:28 K
  Top : PMIOPort  Side=Left
  Bottom : PMIOPort  Port=2  Side=Right
  connections:
  ArrayTop/RConn1 -- Top/RConn1
  Ground_A1R1(LivingRoom)Blk/LConn1 -- ArrayTop/LConn1
  Ground_A1R2(Bedroom)Blk/LConn1 -- ArrayTop/LConn2
  Ground_A1R3(Kitchen)Blk/LConn1 -- ArrayTop/LConn3
  Ground_A1R4(Bathroom)Blk/LConn1 -- ArrayTop/LConn4
  Ground_A1R5(FireExit)Blk/LConn1 -- ArrayTop/LConn5
  ArrayBottom/RConn1 -- Bottom/RConn1
  Ground_A1R1(LivingRoom)Blk/RConn1 -- ArrayBottom/LConn1
  Ground_A1R2(Bedroom)Blk/RConn1 -- ArrayBottom/LConn2
  Ground_A1R3(Kitchen)Blk/RConn1 -- ArrayBottom/LConn3
  Ground_A1R4(Bathroom)Blk/RConn1 -- ArrayBottom/LConn4
  Ground_A1R5(FireExit)Blk/RConn1 -- ArrayBottom/LConn5
